simulink model "test_loopback_buf"  (Simulink 6.2)
settings: Solver=ode45  StartTime=0.0  StopTime=4000  RelTol=1e-3
undefined symbols (not defined in the file): Down, Up
libraries: xbsIndex_r3 x1383, xps_library x52, casper_library x37
(part 8 of 8)

== system test_loopback_buf/xaui_buffer_old/data_FWFT/set_cnt ==
  set : Inport  Port=1  LatchInput=off
  undo : Inport  Port=2  LatchInput=off
  en : Inport  Port=3  LatchInput=off
  Counter4 : xbsIndex_r3/Counter  cnt_type=Free Running  n_bits=depth_bits + 1  bin_pt=0  arith_type=Unsigned  start_count=0  cnt_to=Inf  cnt_by_val=1  operation=Up  explicit_period=on  period=1  load_pin=on  rst=off  en=on  dbl_ovrd=off  show_param=off  use_rpm=on  gen_core=off
      settings: xl_area=[0, 0, 0, 0, 0, 0, 0]
  Inverter : xbsIndex_r3/Inverter  latency=0  explicit_period=off  period=1  en=off  dbl_ovrd=off  show_param=off
      settings: xl_area=[0, 0, 0, 0, 0, 0, 0]
  Inverter1 : xbsIndex_r3/Inverter  latency=0  explicit_period=off  period=1  en=off  dbl_ovrd=off  show_param=off
      settings: xl_area=[0, 0, 0, 0, 0, 0, 0]
  Logical1 : xbsIndex_r3/Logical  logical_function=AND  inputs=3  precision=Full  arith_type=Unsigned  n_bits=8  bin_pt=2  align_bp=on  latency=0  explicit_period=off  period=1  en=off  dbl_ovrd=off  show_param=off
      settings: xl_area=[0, 0, 0, 0, 0, 0, 0]
  Logical4 : xbsIndex_r3/Logical  logical_function=AND  inputs=3  precision=Full  arith_type=Unsigned  n_bits=8  bin_pt=2  align_bp=on  latency=1  explicit_period=off  period=1  en=off  dbl_ovrd=off  show_param=off
      settings: xl_area=[0, 0, 0, 0, 0, 0, 0]
  Register2 : xbsIndex_r3/Register  init=0  reg_only_valid=off  explicit_period=off  period=1  rst=off  en=on  out_en=off  dbl_ovrd=off  show_param=off
      settings: xl_area=[0, 0, 0, 0, 0, 0, 0]
  set_cnt : Outport
  cnt : Outport  Port=2
  wires:
  Inverter1/1 -> Logical1/3
  Inverter/1 -> Logical4/3
  undo/1 -> Inverter/1, Logical1/1
  Logical1/1 -> Counter4/1
  set/1 -> Logical4/1
  Logical4/1 -> Inverter1/1, Register2/2
  Register2/1 -> set_cnt/1, Counter4/2
  en/1 -> Logical4/2, Logical1/2, Counter4/3
  Counter4/1 -> Register2/1, cnt/1

== system test_loopback_buf/xaui_buffer_old/ip_fifo/set_cnt ==
  set : Inport  Port=1  LatchInput=off
  undo : Inport  Port=2  LatchInput=off
  en : Inport  Port=3  LatchInput=off
  Counter4 : xbsIndex_r3/Counter  cnt_type=Free Running  n_bits=depth_bits + 1  bin_pt=0  arith_type=Unsigned  start_count=0  cnt_to=Inf  cnt_by_val=1  operation=Up  explicit_period=on  period=1  load_pin=on  rst=off  en=on  dbl_ovrd=off  show_param=off  use_rpm=on  gen_core=off
      settings: xl_area=[0, 0, 0, 0, 0, 0, 0]
  Inverter : xbsIndex_r3/Inverter  latency=0  explicit_period=off  period=1  en=off  dbl_ovrd=off  show_param=off
      settings: xl_area=[0, 0, 0, 0, 0, 0, 0]
  Inverter1 : xbsIndex_r3/Inverter  latency=0  explicit_period=off  period=1  en=off  dbl_ovrd=off  show_param=off
      settings: xl_area=[0, 0, 0, 0, 0, 0, 0]
  Logical1 : xbsIndex_r3/Logical  logical_function=AND  inputs=3  precision=Full  arith_type=Unsigned  n_bits=8  bin_pt=2  align_bp=on  latency=0  explicit_period=off  period=1  en=off  dbl_ovrd=off  show_param=off
      settings: xl_area=[0, 0, 0, 0, 0, 0, 0]
  Logical4 : xbsIndex_r3/Logical  logical_function=AND  inputs=3  precision=Full  arith_type=Unsigned  n_bits=8  bin_pt=2  align_bp=on  latency=1  explicit_period=off  period=1  en=off  dbl_ovrd=off  show_param=off
      settings: xl_area=[0, 0, 0, 0, 0, 0, 0]
  Register2 : xbsIndex_r3/Register  init=0  reg_only_valid=off  explicit_period=off  period=1  rst=off  en=on  out_en=off  dbl_ovrd=off  show_param=off
      settings: xl_area=[0, 0, 0, 0, 0, 0, 0]
  set_cnt : Outport
  cnt : Outport  Port=2
  wires:
  Inverter1/1 -> Logical1/3
  Inverter/1 -> Logical4/3
  undo/1 -> Inverter/1, Logical1/1
  Logical1/1 -> Counter4/1
  set/1 -> Logical4/1
  Logical4/1 -> Inverter1/1, Register2/2
  Register2/1 -> set_cnt/1, Counter4/2
  en/1 -> Logical4/2, Logical1/2, Counter4/3
  Counter4/1 -> Register2/1, cnt/1

== system test_loopback_buf/xaui_buffer_old1/data_FWFT/set_cnt ==
  set : Inport  Port=1  LatchInput=off
  undo : Inport  Port=2  LatchInput=off
  en : Inport  Port=3  LatchInput=off
  Counter4 : xbsIndex_r3/Counter  cnt_type=Free Running  n_bits=depth_bits + 1  bin_pt=0  arith_type=Unsigned  start_count=0  cnt_to=Inf  cnt_by_val=1  operation=Up  explicit_period=on  period=1  load_pin=on  rst=off  en=on  dbl_ovrd=off  show_param=off  use_rpm=on  gen_core=off
      settings: xl_area=[0, 0, 0, 0, 0, 0, 0]
  Inverter : xbsIndex_r3/Inverter  latency=0  explicit_period=off  period=1  en=off  dbl_ovrd=off  show_param=off
      settings: xl_area=[0, 0, 0, 0, 0, 0, 0]
  Inverter1 : xbsIndex_r3/Inverter  latency=0  explicit_period=off  period=1  en=off  dbl_ovrd=off  show_param=off
      settings: xl_area=[0, 0, 0, 0, 0, 0, 0]
  Logical1 : xbsIndex_r3/Logical  logical_function=AND  inputs=3  precision=Full  arith_type=Unsigned  n_bits=8  bin_pt=2  align_bp=on  latency=0  explicit_period=off  period=1  en=off  dbl_ovrd=off  show_param=off
      settings: xl_area=[0, 0, 0, 0, 0, 0, 0]
  Logical4 : xbsIndex_r3/Logical  logical_function=AND  inputs=3  precision=Full  arith_type=Unsigned  n_bits=8  bin_pt=2  align_bp=on  latency=1  explicit_period=off  period=1  en=off  dbl_ovrd=off  show_param=off
      settings: xl_area=[0, 0, 0, 0, 0, 0, 0]
  Register2 : xbsIndex_r3/Register  init=0  reg_only_valid=off  explicit_period=off  period=1  rst=off  en=on  out_en=off  dbl_ovrd=off  show_param=off
      settings: xl_area=[0, 0, 0, 0, 0, 0, 0]
  set_cnt : Outport
  cnt : Outport  Port=2
  wires:
  Inverter1/1 -> Logical1/3
  Inverter/1 -> Logical4/3
  undo/1 -> Inverter/1, Logical1/1
  Logical1/1 -> Counter4/1
  set/1 -> Logical4/1
  Logical4/1 -> Inverter1/1, Register2/2
  Register2/1 -> set_cnt/1, Counter4/2
  en/1 -> Logical4/2, Logical1/2, Counter4/3
  Counter4/1 -> Register2/1, cnt/1

== system test_loopback_buf/xaui_buffer_old1/ip_fifo/set_cnt ==
  set : Inport  Port=1  LatchInput=off
  undo : Inport  Port=2  LatchInput=off
  en : Inport  Port=3  LatchInput=off
  Counter4 : xbsIndex_r3/Counter  cnt_type=Free Running  n_bits=depth_bits + 1  bin_pt=0  arith_type=Unsigned  start_count=0  cnt_to=Inf  cnt_by_val=1  operation=Up  explicit_period=on  period=1  load_pin=on  rst=off  en=on  dbl_ovrd=off  show_param=off  use_rpm=on  gen_core=off
      settings: xl_area=[0, 0, 0, 0, 0, 0, 0]
  Inverter : xbsIndex_r3/Inverter  latency=0  explicit_period=off  period=1  en=off  dbl_ovrd=off  show_param=off
      settings: xl_area=[0, 0, 0, 0, 0, 0, 0]
  Inverter1 : xbsIndex_r3/Inverter  latency=0  explicit_period=off  period=1  en=off  dbl_ovrd=off  show_param=off
      settings: xl_area=[0, 0, 0, 0, 0, 0, 0]
  Logical1 : xbsIndex_r3/Logical  logical_function=AND  inputs=3  precision=Full  arith_type=Unsigned  n_bits=8  bin_pt=2  align_bp=on  latency=0  explicit_period=off  period=1  en=off  dbl_ovrd=off  show_param=off
      settings: xl_area=[0, 0, 0, 0, 0, 0, 0]
  Logical4 : xbsIndex_r3/Logical  logical_function=AND  inputs=3  precision=Full  arith_type=Unsigned  n_bits=8  bin_pt=2  align_bp=on  latency=1  explicit_period=off  period=1  en=off  dbl_ovrd=off  show_param=off
      settings: xl_area=[0, 0, 0, 0, 0, 0, 0]
  Register2 : xbsIndex_r3/Register  init=0  reg_only_valid=off  explicit_period=off  period=1  rst=off  en=on  out_en=off  dbl_ovrd=off  show_param=off
      settings: xl_area=[0, 0, 0, 0, 0, 0, 0]
  set_cnt : Outport
  cnt : Outport  Port=2
  wires:
  Inverter1/1 -> Logical1/3
  Inverter/1 -> Logical4/3
  undo/1 -> Inverter/1, Logical1/1
  Logical1/1 -> Counter4/1
  set/1 -> Logical4/1
  Logical4/1 -> Inverter1/1, Register2/2
  Register2/1 -> set_cnt/1, Counter4/2
  en/1 -> Logical4/2, Logical1/2, Counter4/3
  Counter4/1 -> Register2/1, cnt/1
